simulink library "rov_design_analysis"  (Simulink 6.0)
settings: Solver=ode45  SolverMode=SingleTasking  StartTime=0.0  StopTime=10.0  RelTol=1e-3
undefined symbols (not defined in the file or in its folder): amp, At, B, Bt, Ct, cycles, D, den, DL, Do, DQ, DQL, freq, frtest, I, L, m, M, Ma, magnitude, MaU, Mt, nmiss, num, phase, rg, sigbuilder_block, slcm, T, W, xb, xg, Xudot, yb, yg, Yvdot, zb, zg, Zwdot
libraries: simulink_extras x32, simulink x27, rov_design_analysis x15, marine_gnc x10, dspmtrx2 x6, dspstat3 x4
(part 5 of 9)

== system rov_design_analysis/ROV Controller /Nonlinear-Sliding-Mode Cascaded  Controller - 6 DoF/Subsystem2 ==
  note: 2nd order
      | dynamic thruster model
  "Input " : Inport  Port=1  LatchInput=off
  Demux1 : Demux
  Mux2 : Mux
  SubSystem11 : Subsystem
  SubSystem12 : Subsystem
  SubSystem5 : Subsystem
  SubSystem6 : Subsystem
  "Output " : Outport
  wires:
  Demux1/1 -> SubSystem12/1(volt)
  SubSystem12/1(thrust) -> Mux2/1
  Demux1/2 -> SubSystem5/1(volt)
  SubSystem5/1(thrust) -> Mux2/2
  SubSystem6/1(thrust) -> Mux2/3
  Demux1/3 -> SubSystem6/1(volt)
  Demux1/4 -> SubSystem11/1(volt)
  SubSystem11/1(thrust) -> Mux2/4
  Mux2/1 -> "Output "/1
  "Input "/1 -> Demux1/1

== system rov_design_analysis/ROV Controller /Nonlinear-Sliding-Mode Cascaded  Controller - 6 DoF/kd ==
  body vel : Inport  Port=1  LatchInput=off
  Demux : Demux  Outputs=6
  Mux : Mux  Inputs=6
  kd1 : Gain  Gain=22  SaturateOnIntegerOverflow=on
  kd2 : Gain  Gain=27  SaturateOnIntegerOverflow=on
  kd3 : Gain  Gain=3  SaturateOnIntegerOverflow=on
  kd4 : Gain  Gain=2.6  SaturateOnIntegerOverflow=on
  kd5 : Gain  Gain=3  SaturateOnIntegerOverflow=on
  kd6 : Gain  Gain=10  SaturateOnIntegerOverflow=on
  kd : Outport
  wires:
  Mux/1 -> kd/1
  body vel/1 -> Demux/1
  Demux/1 -> kd1/1
  Demux/2 -> kd2/1
  Demux/3 -> kd3/1
  Demux/4 -> kd4/1
  Demux/5 -> kd5/1
  Demux/6 -> kd6/1
  kd1/1 -> Mux/1
  kd2/1 -> Mux/2
  kd3/1 -> Mux/3
  kd4/1 -> Mux/4
  kd5/1 -> Mux/5
  kd6/1 -> Mux/6

== system rov_design_analysis/ROV Controller /Nonlinear-Sliding-Mode Cascaded  Controller - 6 DoF/kp  ==
  body vel : Inport  Port=1  LatchInput=off
  Demux : Demux  Outputs=6
  Mux : Mux  Inputs=6
  kp1 : Gain  Gain=111  SaturateOnIntegerOverflow=on
  kp2 : Gain  Gain=200  SaturateOnIntegerOverflow=on
  kp3 : Gain  Gain=120  SaturateOnIntegerOverflow=on
  kp4 : Gain  Gain=4  SaturateOnIntegerOverflow=on
  kp5 : Gain  Gain=2  SaturateOnIntegerOverflow=on
  kp6 : Gain  Gain=10  SaturateOnIntegerOverflow=on
  kp : Outport
  wires:
  Mux/1 -> kp/1
  body vel/1 -> Demux/1
  Demux/1 -> kp1/1
  Demux/2 -> kp2/1
  Demux/3 -> kp3/1
  Demux/4 -> kp4/1
  Demux/5 -> kp5/1
  Demux/6 -> kp6/1
  kp1/1 -> Mux/1
  kp2/1 -> Mux/2
  kp3/1 -> Mux/3
  kp4/1 -> Mux/4
  kp5/1 -> Mux/5
  kp6/1 -> Mux/6

== system rov_design_analysis/ROV Controller /Nonlinear-Sliding-Mode Cascaded  Controller - 6 DoF/pipe tracking profile  (Manual) ==
  Mux : Mux  Inputs=6
  phi : Step  Time=0  After=0  SampleTime=0
  theta : Step  Time=0  After=-50  SampleTime=0
  x : Step  Time=0  After=0  SampleTime=0
  y : Step  Time=0  After=0  SampleTime=0
  yaw : Step  Time=0  After=-1.57  SampleTime=0
  z : Step  Time=0  After=-50  SampleTime=0
  manual : Outport
  wires:
  Mux/1 -> manual/1
  z/1 -> Mux/3
  y/1 -> Mux/2
  x/1 -> Mux/1
  yaw/1 -> Mux/6
  phi/1 -> Mux/4
  theta/1 -> Mux/5

== system rov_design_analysis/ROV Controller /P-Decoupled  Cascaded loop Controller  - 6 DoF/Body-fixed to Earth_fixed Transformation1 ==
  Input earth Velocity : Inport  Port=1  LatchInput=off
  Demux : Demux  Outputs=2
  Demux1 : Demux  Outputs=2
  Intregrator2 : Integrator
  Mux1 : Mux  Inputs=2
  Terminator : Terminator
  Transformation matrix R : Subsystem
      mask Display: disp('Transformation R')
  Transformation matrix T : Subsystem
      mask Display: disp('Transformation T')
  Output body velocities : Outport  InitialOutput=0
  wires:
  Intregrator2/1 -> Demux1/1
  Mux1/1 -> Output body velocities/1, Intregrator2/1
  Input earth Velocity/1 -> Demux/1
  Demux1/1 -> Terminator/1
  Transformation matrix T/1(translational earth velocity) -> Mux1/1
  Transformation matrix R/1(angular earth velocity) -> Mux1/2
  Demux1/2 -> Transformation matrix R/2(angular position), Transformation matrix T/2(angular position)
  Demux/1 -> Transformation matrix T/1(translational body velocity)
  Demux/2 -> Transformation matrix R/1(angular body  velocity)

== system rov_design_analysis/ROV Controller /P-Decoupled  Cascaded loop Controller  - 6 DoF/Body-fixed to Earth_fixed Transformation3 ==
  Input earth Velocity : Inport  Port=1  LatchInput=off
  Demux : Demux  Outputs=2
  Demux1 : Demux  Outputs=2
  Intregrator2 : Integrator
  Mux1 : Mux  Inputs=2
  Terminator : Terminator
  Transformation matrix R : Subsystem
      mask Display: disp('Transformation R')
  Transformation matrix T : Subsystem
      mask Display: disp('Transformation T')
  Output body velocities : Outport  InitialOutput=0
  wires:
  Demux/2 -> Transformation matrix R/1(angular body  velocity)
  Demux/1 -> Transformation matrix T/1(translational body velocity)
  Demux1/2 -> Transformation matrix T/2(angular position), Transformation matrix R/2(angular position)
  Transformation matrix R/1(angular earth velocity) -> Mux1/2
  Transformation matrix T/1(translational earth velocity) -> Mux1/1
  Demux1/1 -> Terminator/1
  Input earth Velocity/1 -> Demux/1
  Mux1/1 -> Intregrator2/1, Output body velocities/1
  Intregrator2/1 -> Demux1/1

== system rov_design_analysis/ROV Controller /P-Decoupled  Cascaded loop Controller  - 6 DoF/Pseudo Inverse (n X n) ==
  In1 : Inport  Port=1  LatchInput=off
  Gain : Gain  Gain=pinv(T)  Multiplication=Matrix(K*u)
  Out1 : Outport
  wires:
  Gain/1 -> Out1/1
  In1/1 -> Gain/1

== system rov_design_analysis/ROV Controller /P-Decoupled  Cascaded loop Controller  - 6 DoF/Subsystem2 ==
  note: 2nd order
      | dynamic thruster model
  "Input " : Inport  Port=1  LatchInput=off
  Demux1 : Demux
  Mux2 : Mux
  SubSystem11 : Subsystem
  SubSystem12 : Subsystem
  SubSystem5 : Subsystem
  SubSystem6 : Subsystem
  "Output " : Outport
  wires:
  Demux1/1 -> SubSystem12/1(volt)
  SubSystem12/1(thrust) -> Mux2/1
  Demux1/2 -> SubSystem5/1(volt)
  SubSystem5/1(thrust) -> Mux2/2
  SubSystem6/1(thrust) -> Mux2/3
  Demux1/3 -> SubSystem6/1(volt)
  Demux1/4 -> SubSystem11/1(volt)
  SubSystem11/1(thrust) -> Mux2/4
  Mux2/1 -> "Output "/1
  "Input "/1 -> Demux1/1

== system rov_design_analysis/ROV Controller /P-Decoupled  Cascaded loop Controller  - 6 DoF/kd ==
  body vel : Inport  Port=1  LatchInput=off
  Demux : Demux  Outputs=6
  Mux : Mux  Inputs=6
  kd1 : Gain  Gain=22  SaturateOnIntegerOverflow=on
  kd2 : Gain  Gain=27  SaturateOnIntegerOverflow=on
  kd3 : Gain  Gain=3  SaturateOnIntegerOverflow=on
  kd4 : Gain  Gain=2.6  SaturateOnIntegerOverflow=on
  kd5 : Gain  Gain=3  SaturateOnIntegerOverflow=on
  kd6 : Gain  Gain=10  SaturateOnIntegerOverflow=on
  kd : Outport
  wires:
  Mux/1 -> kd/1
  body vel/1 -> Demux/1
  Demux/1 -> kd1/1
  Demux/2 -> kd2/1
  Demux/3 -> kd3/1
  Demux/4 -> kd4/1
  Demux/5 -> kd5/1
  Demux/6 -> kd6/1
  kd1/1 -> Mux/1
  kd2/1 -> Mux/2
  kd3/1 -> Mux/3
  kd4/1 -> Mux/4
  kd5/1 -> Mux/5
  kd6/1 -> Mux/6

== system rov_design_analysis/ROV Controller /P-Decoupled  Cascaded loop Controller  - 6 DoF/kp  ==
  body vel : Inport  Port=1  LatchInput=off
  Demux : Demux  Outputs=6
  Mux : Mux  Inputs=6
  kp1 : Gain  Gain=111  SaturateOnIntegerOverflow=on
  kp2 : Gain  Gain=200  SaturateOnIntegerOverflow=on
  kp3 : Gain  Gain=120  SaturateOnIntegerOverflow=on
  kp4 : Gain  Gain=4  SaturateOnIntegerOverflow=on
  kp5 : Gain  Gain=2  SaturateOnIntegerOverflow=on
  kp6 : Gain  Gain=10  SaturateOnIntegerOverflow=on
  kp : Outport
  wires:
  Mux/1 -> kp/1
  body vel/1 -> Demux/1
  Demux/1 -> kp1/1
  Demux/2 -> kp2/1
  Demux/3 -> kp3/1
  Demux/4 -> kp4/1
  Demux/5 -> kp5/1
  Demux/6 -> kp6/1
  kp1/1 -> Mux/1
  kp2/1 -> Mux/2
  kp3/1 -> Mux/3
  kp4/1 -> Mux/4
  kp5/1 -> Mux/5
  kp6/1 -> Mux/6

== system rov_design_analysis/ROV Controller /P-Decoupled  Cascaded loop Controller  - 6 DoF/pipe tracking profile  (Manual) ==
  Mux : Mux  Inputs=6
  phi : Step  Time=0  After=0  SampleTime=0
  theta : Step  Time=0  After=-50  SampleTime=0
  x : Step  Time=0  After=0  SampleTime=0
  y : Step  Time=0  After=0  SampleTime=0
  yaw : Step  Time=0  After=-1.57  SampleTime=0
  z : Step  Time=0  After=-50  SampleTime=0
  manual : Outport
  wires:
  Mux/1 -> manual/1
  z/1 -> Mux/3
  y/1 -> Mux/2
  x/1 -> Mux/1
  yaw/1 -> Mux/6
  phi/1 -> Mux/4
  theta/1 -> Mux/5

== system rov_design_analysis/ROV Controller /P-Decoupled  Single loop Controller - 6 DoF /Body-fixed to Earth_fixed Transformation1 ==
  Input earth Velocity : Inport  Port=1  LatchInput=off
  Demux : Demux  Outputs=2
  Demux1 : Demux  Outputs=2
  Intregrator2 : Integrator
  Mux1 : Mux  Inputs=2
  Terminator : Terminator
  Transformation matrix R : Subsystem
      mask Display: disp('Transformation R')
  Transformation matrix T : Subsystem
      mask Display: disp('Transformation T')
  Output body velocities : Outport  InitialOutput=0
  wires:
  Demux/2 -> Transformation matrix R/1(angular body  velocity)
  Demux/1 -> Transformation matrix T/1(translational body velocity)
  Demux1/2 -> Transformation matrix T/2(angular position), Transformation matrix R/2(angular position)
  Transformation matrix R/1(angular earth velocity) -> Mux1/2
  Transformation matrix T/1(translational earth velocity) -> Mux1/1
  Demux1/1 -> Terminator/1
  Input earth Velocity/1 -> Demux/1
  Mux1/1 -> Intregrator2/1, Output body velocities/1
  Intregrator2/1 -> Demux1/1

== system rov_design_analysis/ROV Controller /P-Decoupled  Single loop Controller - 6 DoF /Body-fixed to Earth_fixed Transformation3 ==
  Input earth Velocity : Inport  Port=1  LatchInput=off
  Demux : Demux  Outputs=2
  Demux1 : Demux  Outputs=2
  Intregrator2 : Integrator
  Mux1 : Mux  Inputs=2
  Terminator : Terminator
  Transformation matrix R : Subsystem
      mask Display: disp('Transformation R')
  Transformation matrix T : Subsystem
      mask Display: disp('Transformation T')
  Output body velocities : Outport  InitialOutput=0
  wires:
  Intregrator2/1 -> Demux1/1
  Mux1/1 -> Output body velocities/1, Intregrator2/1
  Input earth Velocity/1 -> Demux/1
  Demux1/1 -> Terminator/1
  Transformation matrix T/1(translational earth velocity) -> Mux1/1
  Transformation matrix R/1(angular earth velocity) -> Mux1/2
  Demux1/2 -> Transformation matrix R/2(angular position), Transformation matrix T/2(angular position)
  Demux/1 -> Transformation matrix T/1(translational body velocity)
  Demux/2 -> Transformation matrix R/1(angular body  velocity)

== system rov_design_analysis/ROV Controller /P-Decoupled  Single loop Controller - 6 DoF /Pseudo Inverse (n X n) ==
  In1 : Inport  Port=1  LatchInput=off
  Gain : Gain  Gain=pinv(T)  Multiplication=Matrix(K*u)
  Out1 : Outport
  wires:
  In1/1 -> Gain/1
  Gain/1 -> Out1/1

== system rov_design_analysis/ROV Controller /P-Decoupled  Single loop Controller - 6 DoF /Subsystem2 ==
  note: 2nd order
      | dynamic thruster model
  "Input " : Inport  Port=1  LatchInput=off
  Demux1 : Demux
  Mux2 : Mux
  SubSystem11 : Subsystem
  SubSystem12 : Subsystem
  SubSystem5 : Subsystem
  SubSystem6 : Subsystem
  "Output " : Outport
  wires:
  "Input "/1 -> Demux1/1
  Mux2/1 -> "Output "/1
  SubSystem11/1(thrust) -> Mux2/4
  Demux1/4 -> SubSystem11/1(volt)
  Demux1/3 -> SubSystem6/1(volt)
  SubSystem6/1(thrust) -> Mux2/3
  SubSystem5/1(thrust) -> Mux2/2
  Demux1/2 -> SubSystem5/1(volt)
  SubSystem12/1(thrust) -> Mux2/1
  Demux1/1 -> SubSystem12/1(volt)

== system rov_design_analysis/ROV Controller /P-Decoupled  Single loop Controller - 6 DoF /kd ==
  body vel : Inport  Port=1  LatchInput=off
  Demux : Demux  Outputs=6
  Mux : Mux  Inputs=6
  kd1 : Gain  Gain=22  SaturateOnIntegerOverflow=on
  kd2 : Gain  Gain=27  SaturateOnIntegerOverflow=on
  kd3 : Gain  Gain=3  SaturateOnIntegerOverflow=on
  kd4 : Gain  Gain=2.6  SaturateOnIntegerOverflow=on
  kd5 : Gain  Gain=3  SaturateOnIntegerOverflow=on
  kd6 : Gain  Gain=10  SaturateOnIntegerOverflow=on
  kd : Outport
  wires:
  kd6/1 -> Mux/6
  kd5/1 -> Mux/5
  kd4/1 -> Mux/4
  kd3/1 -> Mux/3
  kd2/1 -> Mux/2
  kd1/1 -> Mux/1
  Demux/6 -> kd6/1
  Demux/5 -> kd5/1
  Demux/4 -> kd4/1
  Demux/3 -> kd3/1
  Demux/2 -> kd2/1
  Demux/1 -> kd1/1
  body vel/1 -> Demux/1
  Mux/1 -> kd/1

== system rov_design_analysis/ROV Controller /P-Decoupled  Single loop Controller - 6 DoF /kp  ==
  body vel : Inport  Port=1  LatchInput=off
  Demux : Demux  Outputs=6
  Mux : Mux  Inputs=6
  kp1 : Gain  Gain=111  SaturateOnIntegerOverflow=on
  kp2 : Gain  Gain=200  SaturateOnIntegerOverflow=on
  kp3 : Gain  Gain=120  SaturateOnIntegerOverflow=on
  kp4 : Gain  Gain=4  SaturateOnIntegerOverflow=on
  kp5 : Gain  Gain=2  SaturateOnIntegerOverflow=on
  kp6 : Gain  Gain=10  SaturateOnIntegerOverflow=on
  kp : Outport
  wires:
  kp6/1 -> Mux/6
  kp5/1 -> Mux/5
  kp4/1 -> Mux/4
  kp3/1 -> Mux/3
  kp2/1 -> Mux/2
  kp1/1 -> Mux/1
  Demux/6 -> kp6/1
  Demux/5 -> kp5/1
  Demux/4 -> kp4/1
  Demux/3 -> kp3/1
  Demux/2 -> kp2/1
  Demux/1 -> kp1/1
  body vel/1 -> Demux/1
  Mux/1 -> kp/1

== system rov_design_analysis/ROV Controller /P-Decoupled  Single loop Controller - 6 DoF /pipe tracking profile  (Manual) ==
  Mux : Mux  Inputs=6
  phi : Step  Time=0  After=0  SampleTime=0
  theta : Step  Time=0  After=-50  SampleTime=0
  x : Step  Time=0  After=0  SampleTime=0
  y : Step  Time=0  After=0  SampleTime=0
  yaw : Step  Time=0  After=-1.57  SampleTime=0
  z : Step  Time=0  After=-50  SampleTime=0
  manual : Outport
  wires:
  theta/1 -> Mux/5
  phi/1 -> Mux/4
  yaw/1 -> Mux/6
  x/1 -> Mux/1
  y/1 -> Mux/2
  z/1 -> Mux/3
  Mux/1 -> manual/1

== system rov_design_analysis/ROV Controller /ROV design  in earth fixed frame  PID - 6 DoF/Model Info ==
  EmptySubsystem : Subsystem

== system rov_design_analysis/Thruster  Controller/1. Propeller thrust control - one DoF/Speed control ==
  note: Speed control
  Tref : Inport  Port=1  LatchInput=off
  PID Controller : simulink_extras/Additional Linear/PID Controller  P=10  I=12  D=0
  Shaft Dynamic : Subsystem
  Sum : Sum  Inputs=|+-  SaturateOnIntegerOverflow=on  InputSameDT=on
  first order motor dynamic : Subsystem
  propeller Load Torque : Subsystem
  propeller thruster : Subsystem
  "propeller thruster      " : Subsystem
  Ta : Outport
  Qa : Outport  Port=2
  wires:
  first order motor dynamic/1(Qm) -> Shaft Dynamic/1(Qm)
  Sum/1 -> PID Controller/1
  "propeller thruster      "/1(nref) -> Sum/1
  PID Controller/1 -> first order motor dynamic/1(Qc)
  Shaft Dynamic/1(n) -> propeller thruster/1(n), Sum/2, propeller Load Torque/1(n)
  propeller Load Torque/1(Qa) -> Qa/1, Shaft Dynamic/2(Qa)
  propeller thruster/1(Ta) -> Ta/1
  Tref/1 -> "propeller thruster      "/1(Tref)

== system rov_design_analysis/Thruster  Controller/2. Thruster Allocation- RRC ROV/thruster allocation  ==
  note: vel to volt
  vel : Inport  Port=1  LatchInput=off
  on/off : Inport  Port=2  LatchInput=off
  Atomic Subsystem1 : Subsystem  TreatAsAtomicUnit=on
      mask Display: disp('check x >0, send \n signal to thrusters ')
  Atomic Subsystem2 : Subsystem  TreatAsAtomicUnit=on
      mask Display: disp('check y >0, send \n signal to thrusters ')
  Atomic Subsystem3 : Subsystem  TreatAsAtomicUnit=on
      mask Display: disp('check z >0, send \n signal to thrusters ')
  Atomic Subsystem4 : Subsystem  TreatAsAtomicUnit=on
      mask Display: disp('activate T3')
  Atomic Subsystem5 : Subsystem  TreatAsAtomicUnit=on
      mask Display: disp('activate T4')
  Atomic Subsystem6 : Subsystem  TreatAsAtomicUnit=on
      mask Display: disp('activate T2')
  Atomic Subsystem7 : Subsystem  TreatAsAtomicUnit=on
      mask Display: disp('activate T1')
  Atomic Subsystem8 : Subsystem  TreatAsAtomicUnit=on
      mask Display: disp('check yaw >0, send \n signal to thrusters ')
  Demux : Demux
  Demux1 : Demux
  Gain : Gain  Gain=-1
  Gain1 : Gain  Gain=-1
  Gain2 : Gain  Gain=0
  Gain3 : Gain  Gain=0
  Mux : Mux
  volt : Outport
  wires:
  Demux/1 -> Atomic Subsystem1/1(In2)
  Demux/2 -> Atomic Subsystem2/1(In2)
  Demux/3 -> Atomic Subsystem3/1(In2)
  Atomic Subsystem7/1(Out1) -> Mux/1
  vel/1 -> Demux/1
  Demux/4 -> Atomic Subsystem8/1(In2)
  on/off/1 -> Demux1/1
  Mux/1 -> volt/1
  Atomic Subsystem6/1(Out1) -> Mux/2
  Atomic Subsystem4/1(Out1) -> Mux/3
  Atomic Subsystem5/1(Out1) -> Mux/4
  Atomic Subsystem1/1(<0) -> Atomic Subsystem7/1(1), Atomic Subsystem6/1(In1)
  Atomic Subsystem2/1(<0) -> Atomic Subsystem4/1(In1), Gain/1
  Atomic Subsystem3/1(<0) -> Atomic Subsystem4/2(In2), Atomic Subsystem5/2(In2)
  Gain/1 -> Atomic Subsystem5/1(In1)
  Atomic Subsystem8/1(<0) -> Atomic Subsystem7/2(2), Gain1/1, Gain3/1, Gain2/1
  Gain1/1 -> Atomic Subsystem6/2(In2)
  Gain2/1 -> Atomic Subsystem5/3(In3)
  Demux1/1 -> Atomic Subsystem7/Enable
  Demux1/2 -> Atomic Subsystem6/Enable
  Demux1/3 -> Atomic Subsystem4/Enable
  Demux1/4 -> Atomic Subsystem5/Enable
  Gain3/1 -> Atomic Subsystem4/3(In3)

== system rov_design_analysis/Utilities/Euler Transformation 6 DoF/Transformation matrix R ==
  angular body  velocity : Inport  Port=1  LatchInput=off
  angular position : Inport  Port=2  LatchInput=off
  Mux : Mux  Inputs=3
  Row1 of T : Subsystem
      mask Display: disp('Row 1')
  Row2 of T : Subsystem
      mask Display: disp('Row 2')
  Row3 of T : Subsystem
      mask Display: disp('Row 3')
  angular earth velocity : Outport
  wires:
  angular body  velocity/1 -> Row1 of T/1(angular body  velocity), Row2 of T/1("angular body velocity "), Row3 of T/1("angular body velocity ")
  Row1 of T/1(angular earth velocity (row 1)) -> Mux/1
  Row2 of T/1(angular earth velocity (row 2)) -> Mux/2
  Row3 of T/1(angular earth velocity (row 3)) -> Mux/3
  Mux/1 -> angular earth velocity/1
  angular position/1 -> Row2 of T/2(angular position), Row1 of T/2(angular position), Row3 of T/2(angular position)

== system rov_design_analysis/Utilities/Euler Transformation 6 DoF/Transformation matrix T ==
  translational body velocity : Inport  Port=1  LatchInput=off
  angular position : Inport  Port=2  LatchInput=off
  Mux : Mux  Inputs=3
  Row1 of R : Subsystem
      mask Display: disp('Row 1')
  Row2 of R : Subsystem
      mask Display: disp('Row 2')
  Row3 of R : Subsystem
      mask Display: disp('Row 3')
  translational earth velocity : Outport  InitialOutput=0
  wires:
  translational body velocity/1 -> Row3 of R/1(translational body velocity), Row2 of R/1(translational body velocity), Row1 of R/1(translational body velocity)
  angular position/1 -> Row2 of R/2(angular position), Row1 of R/2(angular position), Row3 of R/2(angular position)
  Row1 of R/1(translational earth velocity (row 1)) -> Mux/1
  Row2 of R/1(translational earth velocity (row 2)) -> Mux/2
  Row3 of R/1(translational earth velocity (row 3)) -> Mux/3
  Mux/1 -> translational earth velocity/1

== system rov_design_analysis/Utilities/Joystrick (4 DoF)/Subsystem ==
  Clock : Clock
      settings: Decimation=10
  Constant : Constant  Value=0
  Constant1 : Constant  Value=slowdown
  S-Function : S-Function  FunctionName=GetJoystick  Parameters=uint8(dzlow),uint8(dzhigh)
  Switch : Switch  Threshold=0.5
  LX : Outport
  LY : Outport  Port=2
  RX : Outport  Port=3
  RY : Outport  Port=4
  RT : Outport  Port=5
  LT : Outport  Port=6
  buttons : Outport  Port=7
  wires:
  Clock/1 -> Switch/1
  Constant/1 -> Switch/3
  S-Function/3 -> RX/1
  S-Function/4 -> RY/1
  S-Function/5 -> RT/1
  S-Function/6 -> LT/1
  S-Function/7 -> buttons/1
  Constant1/1 -> Switch/2
  Switch/1 -> S-Function/1
  S-Function/1 -> LX/1
  S-Function/2 -> LY/1

== system rov_design_analysis/Utilities/Modes indicator-hort/vert/station - 6 DoF/1 ==
  In : Inport  Port=1  LatchInput=off
  Constant1 : Constant  Value=-0.0001
  Constant2 : Constant  Value=0.0001
  Logical Operator : Logic  Operator=OR
  thruster selection - surge : RelationalOperator  Operator=<  InputSameDT=on
  thruster selection - surge1 : RelationalOperator  Operator=>  InputSameDT=on
  Out : Outport
  wires:
  Constant2/1 -> thruster selection - surge1/2
  In/1 -> thruster selection - surge/1, thruster selection - surge1/1
  Logical Operator/1 -> Out/1
  Constant1/1 -> thruster selection - surge/2
  thruster selection - surge1/1 -> Logical Operator/1
  thruster selection - surge/1 -> Logical Operator/2

== system rov_design_analysis/Utilities/Modes indicator-hort/vert/station - 6 DoF/2 ==
  In1 : Inport  Port=1  LatchInput=off
  Constant1 : Constant  Value=-0.0001
  Constant2 : Constant  Value=0.0001
  Logical Operator : Logic  Operator=OR
  thruster selection - surge : RelationalOperator  Operator=<  InputSameDT=on
  thruster selection - surge1 : RelationalOperator  Operator=>  InputSameDT=on
  Out1 : Outport
  wires:
  thruster selection - surge/1 -> Logical Operator/2
  thruster selection - surge1/1 -> Logical Operator/1
  Constant1/1 -> thruster selection - surge/2
  Logical Operator/1 -> Out1/1
  In1/1 -> thruster selection - surge1/1, thruster selection - surge/1
  Constant2/1 -> thruster selection - surge1/2

== system rov_design_analysis/Utilities/Modes indicator-hort/vert/station - 6 DoF/3 ==
  In1 : Inport  Port=1  LatchInput=off
  Constant1 : Constant  Value=-0.0001
  Constant2 : Constant  Value=0.0001
  Logical Operator : Logic  Operator=OR
  thruster selection - surge : RelationalOperator  Operator=<  InputSameDT=on
  thruster selection - surge1 : RelationalOperator  Operator=>  InputSameDT=on
  Out1 : Outport
  wires:
  thruster selection - surge/1 -> Logical Operator/2
  thruster selection - surge1/1 -> Logical Operator/1
  Constant1/1 -> thruster selection - surge/2
  Logical Operator/1 -> Out1/1
  In1/1 -> thruster selection - surge1/1, thruster selection - surge/1
  Constant2/1 -> thruster selection - surge1/2

== system rov_design_analysis/Utilities/Modes indicator-hort/vert/station - 6 DoF/4 ==
  In1 : Inport  Port=1  LatchInput=off
  Constant1 : Constant  Value=-0.0001
  Constant2 : Constant  Value=0.0001
  Logical Operator : Logic  Operator=OR
  thruster selection - surge : RelationalOperator  Operator=<  InputSameDT=on
  thruster selection - surge1 : RelationalOperator  Operator=>  InputSameDT=on
  Out1 : Outport
  wires:
  thruster selection - surge/1 -> Logical Operator/2
  thruster selection - surge1/1 -> Logical Operator/1
  Constant1/1 -> thruster selection - surge/2
  Logical Operator/1 -> Out1/1
  In1/1 -> thruster selection - surge1/1, thruster selection - surge/1
  Constant2/1 -> thruster selection - surge1/2

== system rov_design_analysis/Utilities/Modes indicator-hort/vert/station - 6 DoF/5 ==
  In1 : Inport  Port=1  LatchInput=off
  Constant1 : Constant  Value=-0.0001
  Constant2 : Constant  Value=0.0001
  Logical Operator : Logic  Operator=OR
  thruster selection - surge : RelationalOperator  Operator=<  InputSameDT=on
  thruster selection - surge1 : RelationalOperator  Operator=>  InputSameDT=on
  Out1 : Outport
  wires:
  thruster selection - surge/1 -> Logical Operator/2
  thruster selection - surge1/1 -> Logical Operator/1
  Constant1/1 -> thruster selection - surge/2
  Logical Operator/1 -> Out1/1
  In1/1 -> thruster selection - surge1/1, thruster selection - surge/1
  Constant2/1 -> thruster selection - surge1/2

== system rov_design_analysis/Utilities/Modes indicator-hort/vert/station - 6 DoF/6 ==
  In1 : Inport  Port=1  LatchInput=off
  Constant1 : Constant  Value=-0.0001
  Constant2 : Constant  Value=0.0001
  Logical Operator : Logic  Operator=OR
  thruster selection - surge : RelationalOperator  Operator=<  InputSameDT=on
  thruster selection - surge1 : RelationalOperator  Operator=>  InputSameDT=on
  Out1 : Outport
  wires:
  thruster selection - surge/1 -> Logical Operator/2
  thruster selection - surge1/1 -> Logical Operator/1
  Constant1/1 -> thruster selection - surge/2
  Logical Operator/1 -> Out1/1
  In1/1 -> thruster selection - surge1/1, thruster selection - surge/1
  Constant2/1 -> thruster selection - surge1/2

== system rov_design_analysis/Utilities/Process Capability  (1 DoF)/cpk  ==
  mean : Inport  Port=1  LatchInput=off
  desired : Inport  Port=2  LatchInput=off
  3*sigma : Inport  Orientation=up  Port=3  LatchInput=off
  Divide : Product  Inputs=*/  OutScaling=2^-10
  Divide1 : Product  Inputs=*/  OutScaling=2^-10
  LSL : Gain  Gain=0.9
  MinMax : MinMax  Inputs=2
  Subtract : Sum  Inputs=-+  OutScaling=2^-10
  Subtract1 : Sum  Inputs=+-  OutScaling=2^-10
  "USL " : Gain  Gain=1.1
  cpk : Outport
  wires:
  desired/1 -> LSL/1, "USL "/1
  "USL "/1 -> Subtract/2
  mean/1 -> Subtract1/1, Subtract/1
  Subtract/1 -> Divide/1
  3*sigma/1 -> Divide1/2, Divide/2
  LSL/1 -> Subtract1/2
  Subtract1/1 -> Divide1/1
  Divide/1 -> MinMax/1
  Divide1/1 -> MinMax/2
  MinMax/1 -> cpk/1

== system rov_design_analysis/Utilities/Switching sequence/Signal Builder2 ==
  Demux : Demux  Tag=STV Demux  Outputs=7
  FromWs : FromWorkspace  Tag=STV FromWs  VariableName=tuvar  SampleTime=0  SigBuilderData=DataTag1  VnvData=DataTag2
      SigBuilderData=|
      | channels(1).label = 'Signal 1'
      | channels(1).allXData = {[0 65 65 700]}
      | channels(1).allYData = {[1 1 0 0]}
      | channels(2).label = 'Signal 2'
      | channels(2).allXData = {[0 70 70 150 150 700]}
      | channels(2).allYData = {[0 0 1 1 0 0]}
      | channels(3).label = 'Signal 3'
      | channels(3).allXData = {[0 160 160 230 230 700]}
      | channels(3).allYData = {[0 0 1 1 0 0]}
      | channels(4).label = 'Signal 4'
      | channels(4).allXData = {[0 240 240 290 290 700]}
      | channels(4).allYData = {[0 0 1 1 0 0]}
      | channels(5).label = 'Signal 5'
      | channels(5).allXData = {[0 300 300 350 350 700]}
      | channels(5).allYData = {[0 0 1 1 0 0]}
      | channels(6).label = 'Signal 6'
      | channels(6).allXData = {[0 360 360 400 400 700]}
      | channels(6).allYData = {[0 0 1 1 0 0]}
      | channels(7).label = 'Signal 7'
      | channels(7).allXData = {[0 410 410 548 548 700]}
      | channels(7).allYData = {[0 0 1 1 0 0]}
      | dataSet.timeRange = [0 700]
      | dataSet.name = 'Group 1'
  Signal 1 : Outport  Tag=STV Outport
  Signal 2 : Outport  Tag=STV Outport  Port=2
  Signal 3 : Outport  Tag=STV Outport  Port=3
  Signal 4 : Outport  Tag=STV Outport  Port=4
  Signal 5 : Outport  Tag=STV Outport  Port=5
  Signal 6 : Outport  Tag=STV Outport  Port=6
  Signal 7 : Outport  Tag=STV Outport  Port=7
  wires:
  Demux/1 -> Signal 1/1
  FromWs/1 -> Demux/1
  Demux/2 -> Signal 2/1
  Demux/3 -> Signal 3/1
  Demux/4 -> Signal 4/1
  Demux/5 -> Signal 5/1
  Demux/6 -> Signal 6/1
  Demux/7 -> Signal 7/1

== system rov_design_analysis/Utilities/Z-score (1 DoF)/Zscore  ==
  mean : Inport  Port=1  LatchInput=off
  desired : Inport  Port=2  LatchInput=off
  3*sigma : Inport  Orientation=up  Port=3  LatchInput=off
  Divide : Product  Inputs=*/  OutScaling=2^-10
  Divide1 : Product  Inputs=*/  OutScaling=2^-10
  Gain8 : Gain  Gain=3
  LSL : Gain  Gain=0.9
  MinMax : MinMax  Inputs=2
  Subtract : Sum  Inputs=-+  OutScaling=2^-10
  Subtract1 : Sum  Inputs=+-  OutScaling=2^-10
  "USL " : Gain  Gain=1.1
  Zscore : Outport
  wires:
  MinMax/1 -> Gain8/1
  Divide1/1 -> MinMax/2
  Divide/1 -> MinMax/1
  Subtract1/1 -> Divide1/1
  LSL/1 -> Subtract1/2
  3*sigma/1 -> Divide/2, Divide1/2
  Subtract/1 -> Divide/1
  mean/1 -> Subtract/1, Subtract1/1
  "USL "/1 -> Subtract/2
  desired/1 -> "USL "/1, LSL/1
  Gain8/1 -> Zscore/1

== system rov_design_analysis/Utilities/pipeline  tracking planner  (6 DoF) /coupled input ==
  In : Inport  Orientation=down  Port=1  LatchInput=off
  relative pt : MultiPortSwitch  Inputs=7
  "x25, y=0, z=50 yaw=1.57" : Subsystem
  "x=0,y=0, z=0 yaw=0  " : Subsystem
  "x=0,y=0, z=0 yaw=0  1" : Subsystem
  "x=0,y=0, z=0 yaw=0  2" : Subsystem
  "x=15,y=0, z=45 yaw=0 " : Subsystem
  "x=25,y=40, z=50 yaw=0" : Subsystem
  "x=y=0, z=-50 yaw=0  " : Subsystem
  Out : Outport
  wires:
  "x=y=0, z=-50 yaw=0  "/1(1) -> relative pt/2  "1"
  In/1 -> relative pt/1
  relative pt/1 -> Out/1
  "x=15,y=0, z=45 yaw=0 "/1(2) -> relative pt/3  "2"
  "x25, y=0, z=50 yaw=1.57"/1(3) -> relative pt/4  "3"
  "x=25,y=40, z=50 yaw=0"/1(4) -> relative pt/5  "4"
  "x=0,y=0, z=0 yaw=0  "/1(5) -> relative pt/6  "5"
  "x=0,y=0, z=0 yaw=0  1"/1(6) -> relative pt/7
  "x=0,y=0, z=0 yaw=0  2"/1(0) -> relative pt/8

== system rov_design_analysis/Utilities/pipeline  tracking planner  (6 DoF) /switching input sequence ==
  Add2 : Sum  Inputs=+++++++  OutScaling=2^-10
  decoupled input seq : Subsystem  Tag=STV Subsys  LoadFcn=sigbuilder_block('load');  StartFcn=sigbuilder_block('start');  StopFcn=sigbuilder_block('stop');  ClipboardFcn=sigbuilder_block('clipboard');  mask(Sigbuilder block){}
      mask help: Sigbuilder GUI
      mask init:
      | if ~strcmp(get_param(bdroot(gcbh),'SimulationStatus'),'stopped') tuvar = sigbuilder_block('maskInit'); end
      settings: CopyFcn=sigbuilder_block('copy');  DeleteFcn=sigbuilder_block('delete');  ModelCloseFcn=sigbuilder_block('modelClose');  PreSaveFcn=sigbuilder_block('preSave');  NameChangeFcn=sigbuilder_block('namechange');  OpenFcn=sigbuilder_block('open',[0 19.5 768 499.5 ]);  CloseFcn=sigbuilder_block('close');
      mask Display: plot(0,0,100,100,[10,10,40,40,10],[80,20,20,80,80],[40,10],[50,50], [40,27,10],[65,72,56],[40,25,25,10],[28,28,43,43]);
  " " : Outport
  wires:
  decoupled input seq/1(Signal 1) -> Add2/1
  decoupled input seq/2(Signal 2) -> Add2/2
  decoupled input seq/3(Signal 3) -> Add2/3
  decoupled input seq/4(Signal 4) -> Add2/4
  decoupled input seq/5(Signal 5) -> Add2/5
  decoupled input seq/6(Signal 6) -> Add2/6
  decoupled input seq/7(Signal 7) -> Add2/7
  Add2/1 -> " "/1

== system rov_design_analysis/Identification/Frequency Response Analysis/Model Info1/EmptySubsystem ==

== system rov_design_analysis/Propeller Models/1.  propeller with motor characteristics - 1DoF (account for dynamic variation in ua,up)/motor and propeller dynamic /blade -thrust ==
  speed : Inport  Port=1  LatchInput=off
  up : Inport  Port=2  LatchInput=off
  1/(1+a) : Math  Operator=reciprocal  SaturateOnIntegerOverflow=on
  Abs1 : Abs  SaturateOnIntegerOverflow=on
  Constant : Constant
  D : Constant  Value=0.1
  D^3 : Math  Operator=pow  SaturateOnIntegerOverflow=on
  D^4 : Math  Operator=pow  SaturateOnIntegerOverflow=on
  Product1 : Product  Inputs=3  SaturateOnIntegerOverflow=on  RndMeth=Zero  InputSameDT=on
  Product2 : Product  Inputs=4  SaturateOnIntegerOverflow=on  RndMeth=Zero  InputSameDT=on
  Product3 : Product  Inputs=3  SaturateOnIntegerOverflow=on  RndMeth=Zero  InputSameDT=on
  Product4 : Product  Inputs=3  SaturateOnIntegerOverflow=on  RndMeth=Zero  InputSameDT=on
  Sum4 : Sum  Inputs=|++  SaturateOnIntegerOverflow=on  InputSameDT=on
  Sum5 : Sum  Inputs=|++  SaturateOnIntegerOverflow=on  InputSameDT=on
  a : Constant  Value=pi*0.1^2/4
  alpha_1 : Constant  Value=-0.022
  alpha_2 : Constant  Value=0.04243
  p : Constant  Value=1024
  p1 : Constant  Value=3
  p2 : Constant  Value=4
  Ta : Outport
  wires:
  alpha_2/1 -> Product4/3
  p2/1 -> D^4/2
  D/1 -> D^4/1, D^3/1
  D^4/1 -> Product4/2
  p/1 -> Product4/1, Product2/2
  Product4/1 -> Product3/3
  Product2/1 -> Product1/2
  Product3/1 -> Sum4/2
  Product1/1 -> Sum4/1
  Sum4/1 -> Ta/1
  speed/1 -> Product3/2, Abs1/1
  Abs1/1 -> Product3/1, Product1/1
  up/1 -> Product1/3
  alpha_1/1 -> Product2/4
  D^3/1 -> Product2/3
  p1/1 -> D^3/2
  1/(1+a)/1 -> Product2/1
  Sum5/1 -> 1/(1+a)/1
  a/1 -> Sum5/2
  Constant/1 -> Sum5/1

== system rov_design_analysis/Propeller Models/1.  propeller with motor characteristics - 1DoF (account for dynamic variation in ua,up)/motor and propeller dynamic /blade-thrust  ==
  speed : Inport  Port=1  LatchInput=off
  up : Inport  Port=2  LatchInput=off
  1/(1+a) : Math  Operator=reciprocal  SaturateOnIntegerOverflow=on
  Abs1 : Abs  SaturateOnIntegerOverflow=on
  Constant : Constant
  D : Constant  Value=0.1
  D^3 : Math  Operator=pow  SaturateOnIntegerOverflow=on
  D^4 : Math  Operator=pow  SaturateOnIntegerOverflow=on
  Product1 : Product  Inputs=3  SaturateOnIntegerOverflow=on  RndMeth=Zero  InputSameDT=on
  Product2 : Product  Inputs=4  SaturateOnIntegerOverflow=on  RndMeth=Zero  InputSameDT=on
  Product3 : Product  Inputs=3  SaturateOnIntegerOverflow=on  RndMeth=Zero  InputSameDT=on
  Product4 : Product  Inputs=3  SaturateOnIntegerOverflow=on  RndMeth=Zero  InputSameDT=on
  Sum4 : Sum  Inputs=|++  SaturateOnIntegerOverflow=on  InputSameDT=on
  Sum5 : Sum  Inputs=|++  SaturateOnIntegerOverflow=on  InputSameDT=on
  a : Constant  Value=pi*0.1^2/4
  alpha_1 : Constant  Value=-0.024
  alpha_2 : Constant  Value=0.0132
  p : Constant  Value=1024
  p1 : Constant  Value=3
  p2 : Constant  Value=4
  Ta : Outport
  wires:
  alpha_2/1 -> Product4/3
  p2/1 -> D^4/2
  D/1 -> D^4/1, D^3/1
  D^4/1 -> Product4/2
  p/1 -> Product4/1, Product2/2
  Product4/1 -> Product3/3
  Product2/1 -> Product1/2
  Product3/1 -> Sum4/2
  Product1/1 -> Sum4/1
  Sum4/1 -> Ta/1
  speed/1 -> Product3/2, Abs1/1
  Abs1/1 -> Product3/1, Product1/1
  up/1 -> Product1/3
  alpha_1/1 -> Product2/4
  D^3/1 -> Product2/3
  p1/1 -> D^3/2
  1/(1+a)/1 -> Product2/1
  Sum5/1 -> 1/(1+a)/1
  a/1 -> Sum5/2
  Constant/1 -> Sum5/1

== system rov_design_analysis/Propeller Models/1.  propeller with motor characteristics - 1DoF (account for dynamic variation in ua,up)/motor and propeller dynamic /blade-torque ==
  speed : Inport  Port=1  LatchInput=off
  up : Inport  Port=2  LatchInput=off
  1/(1+a) : Math  Operator=reciprocal  SaturateOnIntegerOverflow=on
  Abs1 : Abs  SaturateOnIntegerOverflow=on
  Constant : Constant
  D : Constant  Value=0.1
  D^4 : Math  Operator=pow  SaturateOnIntegerOverflow=on
  D^5 : Math  Operator=pow  SaturateOnIntegerOverflow=on
  Product1 : Product  Inputs=3  SaturateOnIntegerOverflow=on  RndMeth=Zero  InputSameDT=on
  Product2 : Product  Inputs=4  SaturateOnIntegerOverflow=on  RndMeth=Zero  InputSameDT=on
  Product3 : Product  Inputs=3  SaturateOnIntegerOverflow=on  RndMeth=Zero  InputSameDT=on
  Product4 : Product  Inputs=3  SaturateOnIntegerOverflow=on  RndMeth=Zero  InputSameDT=on
  Sum4 : Sum  Inputs=|++  SaturateOnIntegerOverflow=on  InputSameDT=on
  Sum5 : Sum  Inputs=|++  SaturateOnIntegerOverflow=on  InputSameDT=on
  a : Constant  Value=pi*0.1^2/4
  beta_1 : Constant  Value=-0.01212
  beta_2 : Constant  Value=0.0626
  p : Constant  Value=1024
  p1 : Constant  Value=4
  p2 : Constant  Value=5
  Qa : Outport
  wires:
  p/1 -> Product4/1, Product2/2
  D/1 -> D^5/1, D^4/1
  beta_2/1 -> Product4/3
  p2/1 -> D^5/2
  D^5/1 -> Product4/2
  Product4/1 -> Product3/3
  Sum4/1 -> Qa/1
  speed/1 -> Product3/2, Abs1/1
  Abs1/1 -> Product3/1, Product1/1
  Product3/1 -> Sum4/2
  Product1/1 -> Sum4/1
  up/1 -> Product1/3
  Product2/1 -> Product1/2
  beta_1/1 -> Product2/4
  D^4/1 -> Product2/3
  p1/1 -> D^4/2
  1/(1+a)/1 -> Product2/1
  Sum5/1 -> 1/(1+a)/1
  a/1 -> Sum5/2
  Constant/1 -> Sum5/1

== system rov_design_analysis/Propeller Models/1.  propeller with motor characteristics - 1DoF (account for dynamic variation in ua,up)/motor and propeller dynamic /blade-torque  ==
  speed : Inport  Port=1  LatchInput=off
  up : Inport  Port=2  LatchInput=off
  1/(1+a) : Math  Operator=reciprocal  SaturateOnIntegerOverflow=on
  Abs1 : Abs  SaturateOnIntegerOverflow=on
  Constant : Constant
  D : Constant  Value=0.1
  D^4 : Math  Operator=pow  SaturateOnIntegerOverflow=on
  D^5 : Math  Operator=pow  SaturateOnIntegerOverflow=on
  Product1 : Product  Inputs=3  SaturateOnIntegerOverflow=on  RndMeth=Zero  InputSameDT=on
  Product2 : Product  Inputs=4  SaturateOnIntegerOverflow=on  RndMeth=Zero  InputSameDT=on
  Product3 : Product  Inputs=3  SaturateOnIntegerOverflow=on  RndMeth=Zero  InputSameDT=on
  Product4 : Product  Inputs=3  SaturateOnIntegerOverflow=on  RndMeth=Zero  InputSameDT=on
  Sum4 : Sum  Inputs=|++  SaturateOnIntegerOverflow=on  InputSameDT=on
  Sum5 : Sum  Inputs=|++  SaturateOnIntegerOverflow=on  InputSameDT=on
  a : Constant  Value=pi*0.1^2/4
  beta_1 : Constant  Value=-0.012
  beta_2 : Constant  Value=0.062
  p : Constant  Value=1024
  p1 : Constant  Value=4
  p2 : Constant  Value=5
  Qa : Outport
  wires:
  p/1 -> Product4/1, Product2/2
  D/1 -> D^5/1, D^4/1
  beta_2/1 -> Product4/3
  p2/1 -> D^5/2
  D^5/1 -> Product4/2
  Product4/1 -> Product3/3
  Sum4/1 -> Qa/1
  speed/1 -> Product3/2, Abs1/1
  Abs1/1 -> Product3/1, Product1/1
  Product3/1 -> Sum4/2
  Product1/1 -> Sum4/1
  up/1 -> Product1/3
  Product2/1 -> Product1/2
  beta_1/1 -> Product2/4
  D^4/1 -> Product2/3
  p1/1 -> D^4/2
  1/(1+a)/1 -> Product2/1
  Sum5/1 -> 1/(1+a)/1
  a/1 -> Sum5/2
  Constant/1 -> Sum5/1

== system rov_design_analysis/Propeller Models/2. propeller with motor characteristics - 1DoF (account for ua only)/motor and propeller dynamic /blade -thrust ==
  speed dot : Inport  Port=1  LatchInput=off
  speed : Inport  Port=2  LatchInput=off
  1 : Gain  Gain=800
  1/(1+a) : Math  Operator=reciprocal  SaturateOnIntegerOverflow=on
  1/(1+a)1 : Math  Operator=reciprocal  SaturateOnIntegerOverflow=on
  40 : Gain  Gain=40
  Abs1 : Abs  SaturateOnIntegerOverflow=on
  Constant : Constant  Value=0.01
  Kr : Constant  Value=2.14
  Kr^2 : Math  Operator=pow  SaturateOnIntegerOverflow=on
  Product{1..4} (4 alike) : Product  SaturateOnIntegerOverflow=on  RndMeth=Zero  InputSameDT=on
  Product5 : Product  Inputs=3  SaturateOnIntegerOverflow=on  RndMeth=Zero  InputSameDT=on
  Product6 : Product  Inputs=3  SaturateOnIntegerOverflow=on  RndMeth=Zero  InputSameDT=on
  Sum4 : Sum  Inputs=|++  SaturateOnIntegerOverflow=on  InputSameDT=on
  a : Constant  Value=pi*0.1^2/4
  p : Constant  Value=1024
  p1 : Constant  Value=2
  Ta : Outport
  wires:
  1/(1+a)/1 -> Product2/1
  p1/1 -> Kr^2/2
  Sum4/1 -> Ta/1
  Product1/1 -> Sum4/1
  Product2/1 -> Product1/2
  Constant/1 -> Product5/1
  a/1 -> Product5/2, Product3/1
  p/1 -> Product5/3, Product3/2
  Product5/1 -> Product2/2
  Kr/1 -> 40/1, Kr^2/1
  40/1 -> 1/(1+a)/1
  speed dot/1 -> Product1/1
  speed/1 -> Abs1/1, Product6/2
  Abs1/1 -> Product6/1
  Product6/1 -> Sum4/2
  Product3/1 -> Product4/2
  1/1 -> 1/(1+a)1/1
  1/(1+a)1/1 -> Product4/1
  Kr^2/1 -> 1/1
  Product4/1 -> Product6/3

== system rov_design_analysis/Propeller Models/2. propeller with motor characteristics - 1DoF (account for ua only)/motor and propeller dynamic /blade -thrust1 ==
  speed dot : Inport  Port=1  LatchInput=off
  speed : Inport  Port=2  LatchInput=off
  1 : Gain  Gain=1458
  1/(1+a) : Math  Operator=reciprocal  SaturateOnIntegerOverflow=on
  1/(1+a)1 : Math  Operator=reciprocal  SaturateOnIntegerOverflow=on
  40 : Gain  Gain=54
  Abs1 : Abs  SaturateOnIntegerOverflow=on
  Constant : Constant  Value=0.01
  Kr : Constant  Value=2.14
  Kr^2 : Math  Operator=pow  SaturateOnIntegerOverflow=on
  Product{1..4} (4 alike) : Product  SaturateOnIntegerOverflow=on  RndMeth=Zero  InputSameDT=on
  Product5 : Product  Inputs=3  SaturateOnIntegerOverflow=on  RndMeth=Zero  InputSameDT=on
  Product6 : Product  Inputs=3  SaturateOnIntegerOverflow=on  RndMeth=Zero  InputSameDT=on
  Sum4 : Sum  Inputs=|++  SaturateOnIntegerOverflow=on  InputSameDT=on
  a : Constant  Value=pi*0.1^2/4
  p : Constant  Value=1024
  p1 : Constant  Value=2
  Ta : Outport
  wires:
  1/(1+a)/1 -> Product2/1
  p1/1 -> Kr^2/2
  Sum4/1 -> Ta/1
  Product1/1 -> Sum4/1
  Product2/1 -> Product1/2
  Constant/1 -> Product5/1
  a/1 -> Product5/2, Product3/1
  p/1 -> Product5/3, Product3/2
  Product5/1 -> Product2/2
  Kr/1 -> 40/1, Kr^2/1
  40/1 -> 1/(1+a)/1
  speed dot/1 -> Product1/1
  speed/1 -> Abs1/1, Product6/2
  Abs1/1 -> Product6/1
  Product6/1 -> Sum4/2
  Product3/1 -> Product4/2
  1/1 -> 1/(1+a)1/1
  1/(1+a)1/1 -> Product4/1
  Kr^2/1 -> 1/1
  Product4/1 -> Product6/3

== system rov_design_analysis/Propeller Models/2. propeller with motor characteristics - 1DoF (account for ua only)/motor and propeller dynamic /blade -torque ==
  speed dot : Inport  Port=1  LatchInput=off
  speed : Inport  Port=2  LatchInput=off
  1 : Gain  Gain=800
  1/(1+a) : Math  Operator=reciprocal  SaturateOnIntegerOverflow=on
  1/(1+a)1 : Math  Operator=reciprocal  SaturateOnIntegerOverflow=on
  40 : Gain  Gain=40
  Abs1 : Abs  SaturateOnIntegerOverflow=on
  Constant : Constant  Value=0.01
  D : Constant  Value=0.1
  Kr : Constant  Value=2.14
  Kr^2 : Math  Operator=pow  SaturateOnIntegerOverflow=on
  Product1 : Product  SaturateOnIntegerOverflow=on  RndMeth=Zero  InputSameDT=on
  Product2 : Product  SaturateOnIntegerOverflow=on  RndMeth=Zero  InputSameDT=on
  Product3 : Product  Inputs=3  SaturateOnIntegerOverflow=on  RndMeth=Zero  InputSameDT=on
  Product4 : Product  SaturateOnIntegerOverflow=on  RndMeth=Zero  InputSameDT=on
  Product5 : Product  Inputs=4  SaturateOnIntegerOverflow=on  RndMeth=Zero  InputSameDT=on
  Product6 : Product  Inputs=3  SaturateOnIntegerOverflow=on  RndMeth=Zero  InputSameDT=on
  Sum4 : Sum  Inputs=|++  SaturateOnIntegerOverflow=on  InputSameDT=on
  a : Constant  Value=pi*0.1^2/4
  p : Constant  Value=1024
  p1 : Constant  Value=2
  Qa : Outport
  wires:
  1/(1+a)/1 -> Product2/1
  p1/1 -> Kr^2/2
  Sum4/1 -> Qa/1
  Product1/1 -> Sum4/1
  Product2/1 -> Product1/2
  Constant/1 -> Product5/1
  a/1 -> Product5/2, Product3/1
  p/1 -> Product5/3, Product3/2
  Product5/1 -> Product2/2
  Kr/1 -> 40/1, Kr^2/1
  40/1 -> 1/(1+a)/1
  speed dot/1 -> Product1/1
  speed/1 -> Abs1/1, Product6/2
  Abs1/1 -> Product6/1
  Product6/1 -> Sum4/2
  Product3/1 -> Product4/2
  1/1 -> 1/(1+a)1/1
  1/(1+a)1/1 -> Product4/1
  Kr^2/1 -> 1/1
  Product4/1 -> Product6/3
  D/1 -> Product5/4, Product3/3

== system rov_design_analysis/Propeller Models/2. propeller with motor characteristics - 1DoF (account for ua only)/motor and propeller dynamic /blade -torque1 ==
  speed dot : Inport  Port=1  LatchInput=off
  speed : Inport  Port=2  LatchInput=off
  1 : Gain  Gain=1458
  1/(1+a) : Math  Operator=reciprocal  SaturateOnIntegerOverflow=on
  1/(1+a)1 : Math  Operator=reciprocal  SaturateOnIntegerOverflow=on
  40 : Gain  Gain=54
  Abs1 : Abs  SaturateOnIntegerOverflow=on
  Constant : Constant  Value=0.01
  D : Constant  Value=0.1
  Kr : Constant  Value=2.14
  Kr^2 : Math  Operator=pow  SaturateOnIntegerOverflow=on
  Product1 : Product  SaturateOnIntegerOverflow=on  RndMeth=Zero  InputSameDT=on
  Product2 : Product  SaturateOnIntegerOverflow=on  RndMeth=Zero  InputSameDT=on
  Product3 : Product  Inputs=3  SaturateOnIntegerOverflow=on  RndMeth=Zero  InputSameDT=on
  Product4 : Product  SaturateOnIntegerOverflow=on  RndMeth=Zero  InputSameDT=on
  Product5 : Product  Inputs=4  SaturateOnIntegerOverflow=on  RndMeth=Zero  InputSameDT=on
  Product6 : Product  Inputs=3  SaturateOnIntegerOverflow=on  RndMeth=Zero  InputSameDT=on
  Sum4 : Sum  Inputs=|++  SaturateOnIntegerOverflow=on  InputSameDT=on
  a : Constant  Value=pi*0.1^2/4
  p : Constant  Value=1024
  p1 : Constant  Value=2
  Qa : Outport
  wires:
  1/(1+a)/1 -> Product2/1
  p1/1 -> Kr^2/2
  Sum4/1 -> Qa/1
  Product1/1 -> Sum4/1
  Product2/1 -> Product1/2
  Constant/1 -> Product5/1
  a/1 -> Product5/2, Product3/1
  p/1 -> Product5/3, Product3/2
  Product5/1 -> Product2/2
  Kr/1 -> 40/1, Kr^2/1
  40/1 -> 1/(1+a)/1
  speed dot/1 -> Product1/1
  speed/1 -> Abs1/1, Product6/2
  Abs1/1 -> Product6/1
  Product6/1 -> Sum4/2
  Product3/1 -> Product4/2
  1/1 -> 1/(1+a)1/1
  1/(1+a)1/1 -> Product4/1
  Kr^2/1 -> 1/1
  Product4/1 -> Product6/3
  D/1 -> Product5/4, Product3/3

== system rov_design_analysis/ROV Models/1. Nonlinear RRC ROV- unperturbed (6DoF)/Model Info/EmptySubsystem ==

== system rov_design_analysis/ROV Controller / Hamiltonian  Interconnection-Damping Assignment  - 2 DoF/Model Info/EmptySubsystem ==

== system rov_design_analysis/ROV Controller / Open-loop ROV - 6 DoF/Model Info/EmptySubsystem ==

== system rov_design_analysis/ROV Controller /Adaptive PD  Cascaded  Controller - 6 DoF/Body-fixed to Earth_fixed Transformation1/Transformation matrix R ==
  angular body  velocity : Inport  Port=1  LatchInput=off
  angular position : Inport  Port=2  LatchInput=off
  Mux : Mux  Inputs=3
  Row1 of T : Subsystem
      mask Display: disp('Row 1')
  Row2 of T : Subsystem
      mask Display: disp('Row 2')
  Row3 of T : Subsystem
      mask Display: disp('Row 3')
  angular earth velocity : Outport  InitialOutput=0
  wires:
  angular body  velocity/1 -> Row1 of T/1(angular body  velocity), Row2 of T/1("angular body velocity "), Row3 of T/1("angular body velocity ")
  Row1 of T/1(angular earth velocity (row 1)) -> Mux/1
  Row2 of T/1(angular earth velocity (row 2)) -> Mux/2
  Row3 of T/1(angular earth velocity (row 3)) -> Mux/3
  Mux/1 -> angular earth velocity/1
  angular position/1 -> Row2 of T/2(angular position), Row1 of T/2(angular position), Row3 of T/2(angular position)

== system rov_design_analysis/ROV Controller /Adaptive PD  Cascaded  Controller - 6 DoF/Body-fixed to Earth_fixed Transformation1/Transformation matrix T ==
  translational body velocity : Inport  Port=1  LatchInput=off
  angular position : Inport  Port=2  LatchInput=off
  Mux : Mux  Inputs=3
  Row1 of R : Subsystem
      mask Display: disp('Row 1')
  Row2 of R : Subsystem
      mask Display: disp('Row 2')
  Row3 of R : Subsystem
      mask Display: disp('Row 3')
  translational earth velocity : Outport  InitialOutput=0
  wires:
  translational body velocity/1 -> Row3 of R/1(translational body velocity), Row2 of R/1(translational body velocity), Row1 of R/1(translational body velocity)
  angular position/1 -> Row2 of R/2(angular position), Row1 of R/2(angular position), Row3 of R/2(angular position)
  Row1 of R/1(translational earth velocity (row 1)) -> Mux/1
  Row2 of R/1(translational earth velocity (row 2)) -> Mux/2
  Row3 of R/1(translational earth velocity (row 3)) -> Mux/3
  Mux/1 -> translational earth velocity/1

== system rov_design_analysis/ROV Controller /Adaptive PD  Cascaded  Controller - 6 DoF/Body-fixed to Earth_fixed Transformation3/Transformation matrix R ==
  angular body  velocity : Inport  Port=1  LatchInput=off
  angular position : Inport  Port=2  LatchInput=off
  Mux : Mux  Inputs=3
  Row1 of T : Subsystem
      mask Display: disp('Row 1')
  Row2 of T : Subsystem
      mask Display: disp('Row 2')
  Row3 of T : Subsystem
      mask Display: disp('Row 3')
  angular earth velocity : Outport  InitialOutput=0
  wires:
  angular position/1 -> Row3 of T/2(angular position), Row1 of T/2(angular position), Row2 of T/2(angular position)
  Mux/1 -> angular earth velocity/1
  Row3 of T/1(angular earth velocity (row 3)) -> Mux/3
  Row2 of T/1(angular earth velocity (row 2)) -> Mux/2
  Row1 of T/1(angular earth velocity (row 1)) -> Mux/1
  angular body  velocity/1 -> Row3 of T/1("angular body velocity "), Row2 of T/1("angular body velocity "), Row1 of T/1(angular body  velocity)

== system rov_design_analysis/ROV Controller /Adaptive PD  Cascaded  Controller - 6 DoF/Body-fixed to Earth_fixed Transformation3/Transformation matrix T ==
  translational body velocity : Inport  Port=1  LatchInput=off
  angular position : Inport  Port=2  LatchInput=off
  Mux : Mux  Inputs=3
  Row1 of R : Subsystem
      mask Display: disp('Row 1')
  Row2 of R : Subsystem
      mask Display: disp('Row 2')
  Row3 of R : Subsystem
      mask Display: disp('Row 3')
  translational earth velocity : Outport  InitialOutput=0
  wires:
  Mux/1 -> translational earth velocity/1
  Row3 of R/1(translational earth velocity (row 3)) -> Mux/3
  Row2 of R/1(translational earth velocity (row 2)) -> Mux/2
  Row1 of R/1(translational earth velocity (row 1)) -> Mux/1
  angular position/1 -> Row3 of R/2(angular position), Row1 of R/2(angular position), Row2 of R/2(angular position)
  translational body velocity/1 -> Row1 of R/1(translational body velocity), Row2 of R/1(translational body velocity), Row3 of R/1(translational body velocity)

== system rov_design_analysis/ROV Controller /Adaptive PD  Cascaded  Controller - 6 DoF/Subsystem2/SubSystem11 ==
  volt : Inport  Port=1  LatchInput=off
  Transfer Fcn : TransferFcn  Numerator=[3700 0.037]  Denominator=[0.5 847.5 76000]
  thrust : Outport
  wires:
  volt/1 -> Transfer Fcn/1
  Transfer Fcn/1 -> thrust/1

== system rov_design_analysis/ROV Controller /Adaptive PD  Cascaded  Controller - 6 DoF/Subsystem2/SubSystem12 ==
  volt : Inport  Port=1  LatchInput=off
  Transfer Fcn : TransferFcn  Numerator=[3700 0.037]  Denominator=[0.5 847.5 76000]
  thrust : Outport
  wires:
  volt/1 -> Transfer Fcn/1
  Transfer Fcn/1 -> thrust/1

== system rov_design_analysis/ROV Controller /Adaptive PD  Cascaded  Controller - 6 DoF/Subsystem2/SubSystem5 ==
  volt : Inport  Port=1  LatchInput=off
  Transfer Fcn : TransferFcn  Numerator=[3700 0.037]  Denominator=[0.5 847.5 76000]
  thrust : Outport
  wires:
  volt/1 -> Transfer Fcn/1
  Transfer Fcn/1 -> thrust/1

== system rov_design_analysis/ROV Controller /Adaptive PD  Cascaded  Controller - 6 DoF/Subsystem2/SubSystem6 ==
  volt : Inport  Port=1  LatchInput=off
  Transfer Fcn : TransferFcn  Numerator=[3700 0.037]  Denominator=[0.5 847.5 76000]
  thrust : Outport
  wires:
  volt/1 -> Transfer Fcn/1
  Transfer Fcn/1 -> thrust/1

== system rov_design_analysis/ROV Controller /Hybrid Control- one DoF/Body-fixed to Earth_fixed Transformation1/Transformation matrix R ==
  angular body  velocity : Inport  Port=1  LatchInput=off
  angular position : Inport  Port=2  LatchInput=off
  Mux : Mux  Inputs=3
  Row1 of T : Subsystem
      mask Display: disp('Row 1')
  Row2 of T : Subsystem
      mask Display: disp('Row 2')
  Row3 of T : Subsystem
      mask Display: disp('Row 3')
  angular earth velocity : Outport  InitialOutput=0
  wires:
  angular position/1 -> Row3 of T/2(angular position), Row1 of T/2(angular position), Row2 of T/2(angular position)
  Mux/1 -> angular earth velocity/1
  Row3 of T/1(angular earth velocity (row 3)) -> Mux/3
  Row2 of T/1(angular earth velocity (row 2)) -> Mux/2
  Row1 of T/1(angular earth velocity (row 1)) -> Mux/1
  angular body  velocity/1 -> Row3 of T/1("angular body velocity "), Row2 of T/1("angular body velocity "), Row1 of T/1(angular body  velocity)
